simulink model "closed_loop"
settings: Solver=ode45  StartTime=0.0  StopTime=20  RelTol=1e-3
settings Model: Creator=kadir  LastModifiedBy=Kadir
settings DataIOCC: LimitDataPoints=on  SaveFormat=Array  ReturnWorkspaceOutputs=off
settings OptimizationCC: LifeSpan=inf  SimCompilerOptimization=Off
settings DebuggingCC: MergeDetectMultiDrivingBlocksExec=none  SolverPrmCheckMsg=warning  MultiTaskDSMMsg=warning  MultiTaskCondExecSysMsg=none  FcnCallInpInsideContextMsg=Enable All  FrameProcessingCompatibilityMsg=warning  StrictBusMsg=ErrorOnBusTreatedAsVector  SFUnexpectedBacktrackingDiag=warning  SFNoUnconditionalDefaultTransitionDiag=warning
settings HardwareCC: ProdBitPerPointer=32  ProdLargestAtomicFloat=None  ProdIntDivRoundTo=Undefined  ProdEndianess=Unspecified  ProdWordSize=32  ProdHWDeviceType=32-bit Generic
settings ModelReferenceCC: PropagateSignalLabelsOutOfModel=off
settings SFSimCC: SimUseLocalCustomCode=off
settings RTWCC: RTWUseLocalCustomCode=off  IncludeERTFirstTime=on  RTWCompilerOptimization=Off
settings GRTTargetCC: GeneratePreprocessorConditionals=Disable all

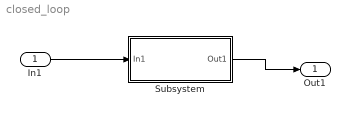
== system closed_loop ==
  In1 : Inport
  Subsystem : Subsystem
  Out1 : Outport
  wires:
  Subsystem/1(Out1) -> Out1/1
  In1/1 -> Subsystem/1(In1)

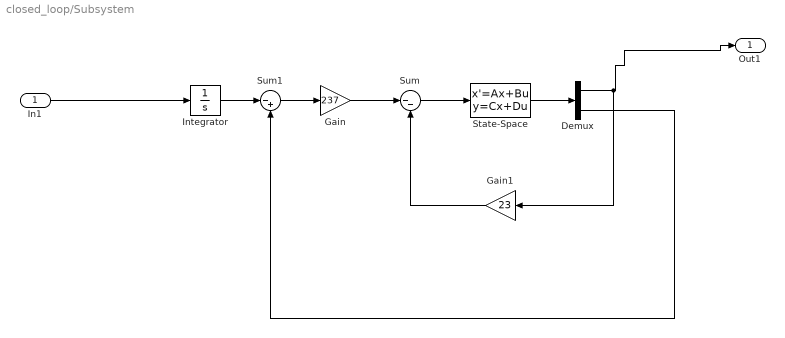
== system closed_loop/Subsystem ==
  In1 : Inport
  Demux : Demux  Outputs=2
  Gain : Gain  Gain=237
  Gain1 : Gain  Gain=23
  Integrator : Integrator
  State-Space : StateSpace  A=[-0.1333 0;1 0]  B=[0.6667 0]'  C=[1 0; 0 1]  D=[0 0]'  X0=[0 0]
  Sum : Sum  Inputs=|--
  Sum1 : Sum  Inputs=|-+
  Out1 : Outport
  wires:
  Sum/1 -> State-Space/1
  Gain/1 -> Sum/1
  State-Space/1 -> Demux/1
  Demux/1 -> Gain1/1, Out1/1
  Gain1/1 -> Sum/2
  Demux/2 -> Sum1/2
  In1/1 -> Integrator/1
  Integrator/1 -> Sum1/1
  Sum1/1 -> Gain/1
